simulink subsystem "MyPiero"  (R2022b)
settings: Solver=VariableStepAuto  StartTime=0.0  StopTime=10.0  RelTol=1e-3
settings Model: Creator=Usuario  LastModifiedBy=Usuario
settings OptimizationCC: ReuseModelBlockBuffer=on
settings RTWCC: GPUComputeCapability=5.0

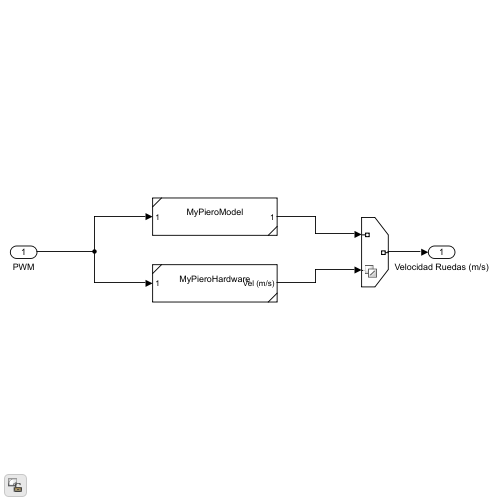
[thumbnail: Simulink's stored preview of the top-level diagram]
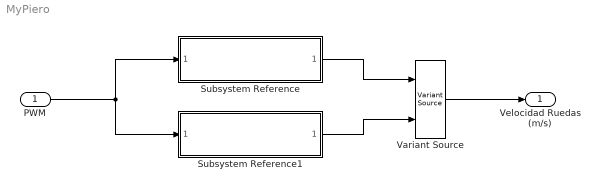
== system MyPiero ==
  PWM : Inport
  Subsystem Reference : Subsystem  ReferencedSubsystem=MyPieroModel
  Subsystem Reference1 : Subsystem  ReferencedSubsystem=MyPieroHardware
  Variant Source : VariantSource  VariantControlMode=sim codegen switching
  Velocidad Ruedas (m/s) : Outport
  wires:
  PWM/1 -> Subsystem Reference/1, Subsystem Reference1/1
  Subsystem Reference/1 -> Variant Source/1
  Subsystem Reference1/1 -> Variant Source/2
  Variant Source/1 -> Velocidad Ruedas (m/s)/1
